simulink model "lab2"  (R2024b)
settings: Solver=ode1  StartTime=0.0  StopTime=10.0  FixedStep=0.001  RelTol=1e-3
settings Model: Creator=maciejklossek  LastModifiedBy=maciejklossek

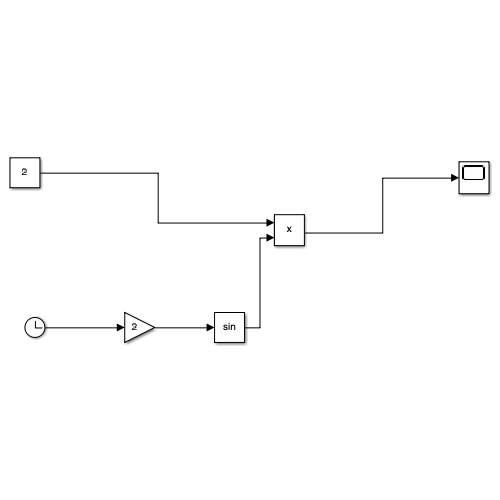
[thumbnail: Simulink's stored preview of the top-level diagram]
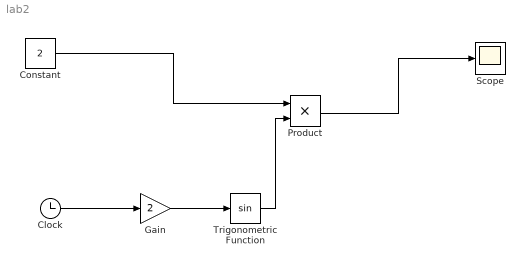
== system lab2 ==
  Clock : Clock
  Constant : Constant  Value=2
  Gain : Gain  Gain=2
  Product : Product
  Scope : Scope
  Trigonometric Function : Trigonometry
  wires:
  Constant/1 -> Product/1
  Trigonometric Function/1 -> Product/2
  Clock/1 -> Gain/1
  Gain/1 -> Trigonometric Function/1
  Product/1 -> Scope/1
